simulink model "regulering_model"  (R2019b)
settings: Solver=VariableStepAuto  StartTime=0.0  StopTime=4000  FixedStep=1  MaxStep=1  RelTol=1e-3
settings Model: Creator=oskar  LastModifiedBy=oskar

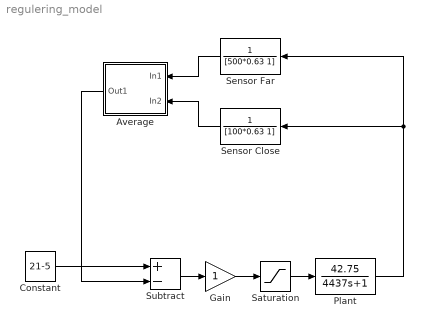
== system regulering_model ==
  Average : Subsystem
  Constant : Constant  Value=21-5
  Gain : Gain
  Plant : TransferFcn  Numerator=[42.75]  Denominator=[4437 1]
  Saturation : Saturate  UpperLimit=1  LowerLimit=0
  Sensor Close : TransferFcn  Denominator=[100*0.63 1]
  Sensor Far : TransferFcn  Denominator=[500*0.63 1]
  Subtract : Sum  Inputs=+-
  wires:
  Constant/1 -> Subtract/1
  Subtract/1 -> Gain/1
  Gain/1 -> Saturation/1
  Saturation/1 -> Plant/1
  Plant/1 -> Sensor Far/1, Sensor Close/1
  Sensor Far/1 -> Average/1(In1)
  Sensor Close/1 -> Average/2(In2)
  Average/1(Out1) -> Subtract/2

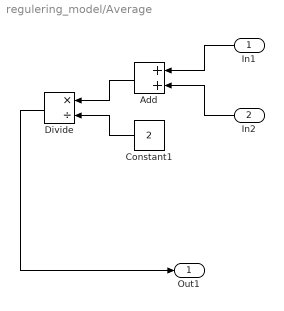
== system regulering_model/Average ==
  In1 : Inport
  In2 : Inport  Port=2
  Add : Sum
  Constant1 : Constant  Value=2
  Divide : Product  Inputs=*/
  Out1 : Outport
  wires:
  Constant1/1 -> Divide/2
  Add/1 -> Divide/1
  In2/1 -> Add/2
  Divide/1 -> Out1/1
  In1/1 -> Add/1
